simulink model "sh_water_supply_system"  (R2019a)
settings: Solver=VariableStepAuto  StartTime=0.0  StopTime=200  MaxStep=0.1  RelTol=1e-3  EnableMultiTasking=on
PreLoadFcn:
  | sh_water_supply_system_init
libraries: sh_lib x35, fl_lib x12, nesl_utility x11
CloseFcn:
  | try,close(h1_sh_water_supply_system),end
  | clear h1_sh_water_supply_system
  | 
  | 
  | clear simlog_sh_water_supply_system
Description:
  | Water Supply System
  | 
  | Copyright 2008-2019 The MathWorks, Inc.
settings Model: Creator=MathWorks  LastModifiedBy=jaych
settings DataIOCC: LimitDataPoints=on  MaxDataPoints=10000  SaveFormat=Array  SignalLoggingSaveFormat=ModelDataLogs  ReturnWorkspaceOutputs=off  SignalLoggingName=logsout_sh_water_supply_system
settings OptimizationCC: ExpressionDepthLimit=2147483647  LifeSpan=inf
settings DebuggingCC: UnderspecifiedInitializationDetection=Classic  MergeDetectMultiDrivingBlocksExec=none  SolverPrmCheckMsg=warning  FcnCallInpInsideContextMsg=warning  AllowSymbolicDim=off  StateNameClashWarn=warning  PregeneratedLibrarySubsystemCodeDiagnostic=none  SFUnexpectedBacktrackingDiag=warning  SFNoUnconditionalDefaultTransitionDiag=warning  SFExecutionAtInitializationDiag=none  ArithmeticOperatorsInVariantConditions=warning
settings HardwareCC: ProdBitPerPointer=32  ProdBitPerSizeT=32  ProdBitPerPtrDiffT=32  ProdLargestAtomicFloat=None  ProdIntDivRoundTo=Undefined  ProdEndianess=Unspecified  ProdWordSize=32  ProdHWDeviceType=32-bit Generic
settings ModelReferenceCC: PropagateSignalLabelsOutOfModel=off
settings SFSimCC: SimUseLocalCustomCode=off
settings RTWCC: RTWUseLocalCustomCode=off
settings CodeAppCC: StateflowObjectComments=on
settings GRTTargetCC: TargetLangStandard=C89/C90 (ANSI)  GeneratePreprocessorConditionals=Disable all  CombineOutputUpdateFcns=off  GRTInterface=on
settings ConfigComp: CovMetricSettings=dw  CovHtmlReporting=on  CovSaveCumulativeToWorkspaceVar=on  CovSaveSingleToWorkspaceVar=on  CovExternalEMLEnable=off  CovSFcnEnable=off
settings SimscapeCC: SimscapeLogType=all  SimscapeLogSimulationStatistics=on  SimscapeLogName=simlog_sh_water_supply_system  SimscapeLogDataHistory=10000

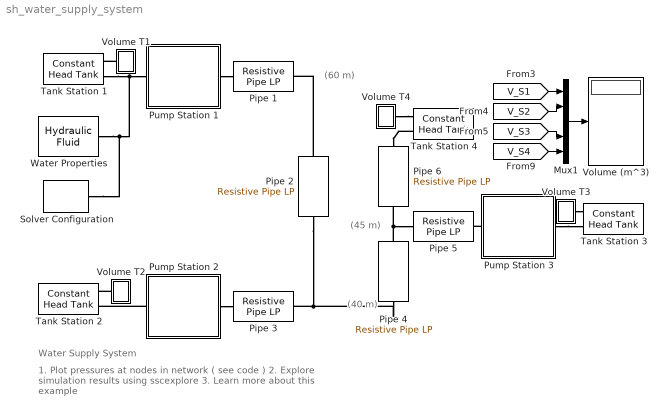
== system sh_water_supply_system ==
  note: (60 m)
  note: (40 m)
  note: (45 m)
  note: Water Supply System
  note: 1. Plot pressures at nodes in network ( see code )
      | 2. Explore simulation results using sscexplore
      | 3. Learn more about this example
  Mux1 : Mux  Inputs=5
  Pipe 1 : sh_lib/Low-Pressure Blocks/Resistive Pipe LP  cs_type=1  d_in=LP_1.diameter mm  area=1e-04 m^2  D_h=0.0112 m  s_factor=64  length=LP_1.length m  length_ad=1 m  roughness=0.005 mm  Re_lam=2e+03  Re_turb=4e+03  elevation_A=LP_1.elevation_A m  elevation_B=LP_1.elevation_B m  g=9.80665 m/s^2  pressure_drop_specify=off  pressure_drop_priority=None  pressure_drop=0 Pa  pressure_drop_nominal_specify=off  pressure_drop_nominal_unit=Pa  pressure_drop_nominal_value=1  flow_rate_specify=off  flow_rate_priority=None  flow_rate=0 m^3/s  flow_rate_nominal_specify=off  flow_rate_nominal_unit=m^3/s  flow_rate_nominal_value=1
      settings: SourceProductName=Simscape Fluids  SourceProductBaseCode=SH
  Pipe 2 : sh_lib/Low-Pressure Blocks/Resistive Pipe LP  cs_type=1  d_in=LP_2.diameter mm  area=1e-04 m^2  D_h=0.0112 m  s_factor=64  length=LP_2.length m  length_ad=1 m  roughness=0.005 mm  Re_lam=2e+03  Re_turb=4e+03  elevation_A=LP_2.elevation_A m  elevation_B=LP_2.elevation_B m  g=9.80665 m/s^2  pressure_drop_specify=off  pressure_drop_priority=None  pressure_drop=0 Pa  pressure_drop_nominal_specify=off  pressure_drop_nominal_unit=Pa  pressure_drop_nominal_value=1  flow_rate_specify=off  flow_rate_priority=None  flow_rate=0 m^3/s  flow_rate_nominal_specify=off  flow_rate_nominal_unit=m^3/s  flow_rate_nominal_value=1
      settings: SourceProductName=Simscape Fluids  SourceProductBaseCode=SH
  Pipe 3 : sh_lib/Low-Pressure Blocks/Resistive Pipe LP  cs_type=1  d_in=LP_3.diameter mm  area=1e-04 m^2  D_h=0.0112 m  s_factor=64  length=LP_3.length m  length_ad=1 m  roughness=0.005 mm  Re_lam=2e+03  Re_turb=4e+03  elevation_A=LP_3.elevation_A m  elevation_B=LP_3.elevation_B m  g=9.80665 m/s^2  pressure_drop_specify=off  pressure_drop_priority=None  pressure_drop=0 Pa  pressure_drop_nominal_specify=off  pressure_drop_nominal_unit=Pa  pressure_drop_nominal_value=1  flow_rate_specify=off  flow_rate_priority=None  flow_rate=0 m^3/s  flow_rate_nominal_specify=off  flow_rate_nominal_unit=m^3/s  flow_rate_nominal_value=1
      settings: SourceProductName=Simscape Fluids  SourceProductBaseCode=SH
  Pipe 4 : sh_lib/Low-Pressure Blocks/Resistive Pipe LP  cs_type=1  d_in=LP_4.diameter mm  area=1e-04 m^2  D_h=0.0112 m  s_factor=64  length=LP_4.length m  length_ad=1 m  roughness=0.005 mm  Re_lam=2e+03  Re_turb=4e+03  elevation_A=LP_4.elevation_A m  elevation_B=LP_4.elevation_B m  g=9.80665 m/s^2  pressure_drop_specify=off  pressure_drop_priority=None  pressure_drop=0 Pa  pressure_drop_nominal_specify=off  pressure_drop_nominal_unit=Pa  pressure_drop_nominal_value=1  flow_rate_specify=off  flow_rate_priority=None  flow_rate=0 m^3/s  flow_rate_nominal_specify=off  flow_rate_nominal_unit=m^3/s  flow_rate_nominal_value=1
      settings: SourceProductName=Simscape Fluids  SourceProductBaseCode=SH
  Pipe 5 : sh_lib/Low-Pressure Blocks/Resistive Pipe LP  cs_type=1  d_in=LP_5.diameter mm  area=1e-04 m^2  D_h=0.0112 m  s_factor=64  length=LP_5.length m  length_ad=1 m  roughness=0.005 mm  Re_lam=2e+03  Re_turb=4e+03  elevation_A=LP_5.elevation_A m  elevation_B=LP_5.elevation_B m  g=9.80665 m/s^2  pressure_drop_specify=off  pressure_drop_priority=None  pressure_drop=0 Pa  pressure_drop_nominal_specify=off  pressure_drop_nominal_unit=Pa  pressure_drop_nominal_value=1  flow_rate_specify=off  flow_rate_priority=None  flow_rate=0 m^3/s  flow_rate_nominal_specify=off  flow_rate_nominal_unit=m^3/s  flow_rate_nominal_value=1
      settings: SourceProductName=Simscape Fluids  SourceProductBaseCode=SH
  Pipe 6 : sh_lib/Low-Pressure Blocks/Resistive Pipe LP  cs_type=1  d_in=LP_6.diameter mm  area=1e-04 m^2  D_h=0.0112 m  s_factor=64  length=LP_6.length m  length_ad=1 m  roughness=0.005 mm  Re_lam=2e+03  Re_turb=4e+03  elevation_A=LP_6.elevation_A m  elevation_B=LP_6.elevation_B m  g=9.80665 m/s^2  pressure_drop_specify=off  pressure_drop_priority=None  pressure_drop=0 Pa  pressure_drop_nominal_specify=off  pressure_drop_nominal_unit=Pa  pressure_drop_nominal_value=1  flow_rate_specify=off  flow_rate_priority=None  flow_rate=0 m^3/s  flow_rate_nominal_specify=off  flow_rate_nominal_unit=m^3/s  flow_rate_nominal_value=1
      settings: SourceProductName=Simscape Fluids  SourceProductBaseCode=SH
  Pump Station 1 : Subsystem  Tag=PublishSubsystem
      mask Display:
      | plot(sin(0:0.5:4.5*pi)*0.9, cos(0:0.5:4.5*pi)*0.9+1.5)
      | plot(sin(0:0.5:4.5*pi)*0.5, cos(0:0.5:4.5*pi)*0.5+1.5)
      | plot(sin(0:0.5:4.5*pi)*0.9, cos(0:0.5:4.5*pi)*0.9-1.5)
      | plot(sin(0:0.5:4.5*pi)*0.5, cos(0:0.5:4.5*pi)*0.5-1.5)
      | 
      | plot([0 -0.9],[1.5 1.5-0.9])
      | plot([0 -0.9],[1.5 1.5-0.9]*-1)
      | 
      | plot([0.45 0.45 0.325 0.325]*2,[1.5 1.5-1.0 1.5-1.0 1.5-0.55])
      | plot([0.45 0.45 0.325 0.325]*2,[1.5 1.5-0.9 1.5-0.9 1.5-0.55]*-1)
      | 
      | plot([2.2 0.95]*-1,[0 0])
      | plot([2.2 0.95],[0 0])
      | 
      | plot([0.95 0.95]*-1,[-0.6 0.6])
      | plot([0.8 0.8],[-0.55 0.55])
      | 
      | 
      | color('white');plot(-3,-2.5);plot(3,2.5);
      | color('red');
      | port_label('LConn',1,'T');
      | port_label('RConn',1,'P');
  Pump Station 2 : Subsystem
      mask Display:
      | %text(0.1,0.7,'Pump Station 1');
      | %text(0.1,0.3,'Elevation 45 m');
      | plot(sin(0:0.5:4.5*pi)*0.9, cos(0:0.5:4.5*pi)*0.9+1.5)
      | plot(sin(0:0.5:4.5*pi)*0.5, cos(0:0.5:4.5*pi)*0.5+1.5)
      | plot(sin(0:0.5:4.5*pi)*0.9, cos(0:0.5:4.5*pi)*0.9-1.5)
      | plot(sin(0:0.5:4.5*pi)*0.5, cos(0:0.5:4.5*pi)*0.5-1.5)
      | 
      | plot([0 -0.9],[1.5 1.5-0.9])
      | plot([0 -0.9],[1.5 1.5-0.9]*-1)
      | 
      | plot([0.45 0.45 0.325 0.325]*2,[1.5 1.5-1.0 1.5-1.0 1.5-0.55])
      | plot([0.45 0.45 0.325 0.325]*2,[1.5 1.5-0.9 1.5-0.9 1.5-0.55]*-1)
      | 
      | plot([2.2 0.95]*-1,[0 0])
      | plot([2.2 0.95],[0 0])
      | 
      | plot([0.95 0.95]*-1,[-0.6 0.6])
      | plot([0.8 0.8],[-0.55 0.55])
      | 
      | 
      | color('white');plot(-3,-2.5);plot(3,2.5);
      | color('red');
      | port_label('LConn',1,'T');
      | port_label('RConn',1,'P');
  Pump Station 3 : Subsystem
      mask Display:
      | %text(0.1,0.7,'Pump Station 1');
      | %text(0.1,0.3,'Elevation 45 m');
      | plot(sin(0:0.5:4.5*pi)*0.9, cos(0:0.5:4.5*pi)*0.9+1.5)
      | plot(sin(0:0.5:4.5*pi)*0.5, cos(0:0.5:4.5*pi)*0.5+1.5)
      | plot(sin(0:0.5:4.5*pi)*0.9, cos(0:0.5:4.5*pi)*0.9-1.5)
      | plot(sin(0:0.5:4.5*pi)*0.5, cos(0:0.5:4.5*pi)*0.5-1.5)
      | 
      | plot([0 -0.9],[1.5 1.5-0.9])
      | plot([0 -0.9],[1.5 1.5-0.9]*-1)
      | 
      | plot([0.45 0.45 0.325 0.325]*2,[1.5 1.5-1.0 1.5-1.0 1.5-0.55])
      | plot([0.45 0.45 0.325 0.325]*2,[1.5 1.5-0.9 1.5-0.9 1.5-0.55]*-1)
      | 
      | plot([2.2 0.95]*-1,[0 0])
      | plot([2.2 0.95],[0 0])
      | 
      | plot([0.95 0.95]*-1,[-0.6 0.6])
      | plot([0.8 0.8],[-0.55 0.55])
      | 
      | 
      | color('white');plot(-3,-2.5);plot(3,2.5);
      | color('red');
      | port_label('LConn',1,'T');
      | port_label('RConn',1,'P');
  Solver Configuration : nesl_utility/Solver Configuration  PhysicalDomain=network_engine_domain  SubClassName=solver  LeftPortType=input  RightPortType=generic  Tones=[]  Harmonics=[]  SimulateNoise=off  Profile=off  UseLocalSampling=off  EnableSwitchedLinearOptims=on  FrequencyDomain=off  UseCCode=off  RelTol=0.001  AbsTol=1e-06  MinStep=1e-09  ToWorkspace=off  RevertToSquareIcSolve=off  NumHomotopyIterations=100  PhasorMode=off  PhasorModeNumHarmonics=1  DoDC=off  ResidualTolerance=1e-9  UseLocalSolver=off  LocalSolverChoice=NE_BACKWARD_EULER_ADVANCER  LocalSolverSampleTime=.001  DoFixedCost=off  MaxNonlinIter=3  MaxModeIter=2  LinearAlgebra=auto  EquationFormulation=NE_TIME_EF  DelaysMemoryBudget=1024  AutomaticFiltering=on  FilteringTimeConstant=0.001  PartitionStorageMethod=AS_NEEDED  PartitionMemoryBudget=1024  PartitionMethod=FAST
  Tank Station 1 : sh_lib/Low-Pressure Blocks/Constant Head Tank  press=0 Pa  fluid_level=station_1.fluid_level m  pipe_diam=0.02 m  loss_coeff=1.2  g=9.80665 m/s^2  volume_specify=on  volume_priority=High  volume=100 m^3  volume_nominal_specify=off  volume_nominal_unit=m^3  volume_nominal_value=1
      settings: SourceProductName=Simscape Fluids  SourceProductBaseCode=SH
  Tank Station 2 : sh_lib/Low-Pressure Blocks/Constant Head Tank  press=0 Pa  fluid_level=station_2.fluid_level m  pipe_diam=0.02 m  loss_coeff=1.2  g=9.80665 m/s^2  volume_specify=on  volume_priority=High  volume=100 m^3  volume_nominal_specify=off  volume_nominal_unit=m^3  volume_nominal_value=1
      settings: SourceProductName=Simscape Fluids  SourceProductBaseCode=SH
  Tank Station 3 : sh_lib/Low-Pressure Blocks/Constant Head Tank  press=0 Pa  fluid_level=station_3.fluid_level m  pipe_diam=0.02 m  loss_coeff=1.2  g=9.80665 m/s^2  volume_specify=on  volume_priority=High  volume=100 m^3  volume_nominal_specify=off  volume_nominal_unit=m^3  volume_nominal_value=1
      settings: SourceProductName=Simscape Fluids  SourceProductBaseCode=SH
  Tank Station 4 : sh_lib/Low-Pressure Blocks/Constant Head Tank  press=0 Pa  fluid_level=0 m  pipe_diam=0.02 m  loss_coeff=1.2  g=9.80665 m/s^2  volume_specify=on  volume_priority=High  volume=0 m^3  volume_nominal_specify=off  volume_nominal_unit=m^3  volume_nominal_value=1
      settings: SourceProductName=Simscape Fluids  SourceProductBaseCode=SH
  Volume (m^3) : Display
  Volume T1 : Subsystem
  Volume T2 : Subsystem
  Volume T3 : Subsystem
  Volume T4 : Subsystem
  Water Properties : sh_lib/Hydraulic Utilities/Hydraulic Fluid  DataSource=1  SelFluid=24  SysTemp=1  TrapAir=0.001  ViscDerFactor=1  range_error=2
      settings: SourceProductName=Simscape Fluids
  wires:
  [V_S1] -> Mux1/1
  [V_S2] -> Mux1/2
  [V_S3] -> Mux1/4
  Mux1/1 -> Volume (m^3)/1
  [V_S4] -> Mux1/5
  connections:
  Pump Station 1/RConn1 -- Pipe 1/LConn1
  Pipe 2/LConn1 -- Pipe 1/RConn1
  Pump Station 2/RConn1 -- Pipe 3/LConn1
  Pipe 4/LConn1 -- Pipe 2/RConn1 -- Pipe 3/RConn1
  Tank Station 4/RConn2 -- Pipe 6/RConn1
  Pipe 4/RConn1 -- Pipe 5/RConn1 -- Pipe 6/LConn1
  Tank Station 1/RConn2 -- Solver Configuration/RConn1 -- Water Properties/RConn1 -- Pump Station 1/LConn1
  Volume T1/LConn1 -- Tank Station 1/RConn1
  Pump Station 2/LConn1 -- Tank Station 2/RConn2
  Volume T2/LConn1 -- Tank Station 2/RConn1
  Pump Station 3/RConn1 -- Pipe 5/LConn1
  Pump Station 3/LConn1 -- Tank Station 3/RConn2
  Volume T3/LConn1 -- Tank Station 3/RConn1
  Volume T4/LConn1 -- Tank Station 4/RConn1

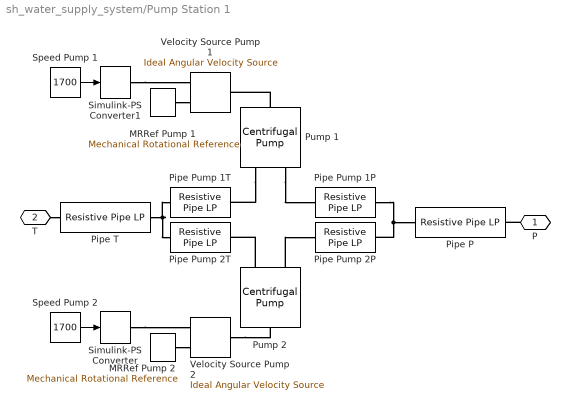
== system sh_water_supply_system/Pump Station 1 ==
  MRRef Pump 1 : fl_lib/Mechanical/Rotational Elements/Mechanical Rotational Reference
  MRRef Pump 2 : fl_lib/Mechanical/Rotational Elements/Mechanical Rotational Reference
  Pipe P : sh_lib/Low-Pressure Blocks/Resistive Pipe LP  cs_type=1  d_in=station_1.pipe_diameter mm  area=1e-04 m^2  D_h=0.0112 m  s_factor=64  length=station_1.pipe_length_3 m  length_ad=1 m  roughness=0.005 mm  Re_lam=2e+03  Re_turb=4e+03  elevation_A=station_1.elevation m  elevation_B=station_1.elevation m  g=9.80665 m/s^2  pressure_drop_specify=off  pressure_drop_priority=None  pressure_drop=0 Pa  pressure_drop_nominal_specify=off  pressure_drop_nominal_unit=Pa  pressure_drop_nominal_value=1  flow_rate_specify=off  flow_rate_priority=None  flow_rate=0 m^3/s  flow_rate_nominal_specify=off  flow_rate_nominal_unit=m^3/s  flow_rate_nominal_value=1
      settings: SourceProductName=Simscape Fluids  SourceProductBaseCode=SH
  Pipe Pump 1P : sh_lib/Low-Pressure Blocks/Resistive Pipe LP  cs_type=1  d_in=station_1.pipe_diameter mm  area=1e-04 m^2  D_h=0.0112 m  s_factor=64  length=station_1.pipe_length_2 m  length_ad=1 m  roughness=0.005 mm  Re_lam=2e+03  Re_turb=4e+03  elevation_A=station_1.elevation m  elevation_B=station_1.elevation m  g=9.80665 m/s^2  pressure_drop_specify=off  pressure_drop_priority=None  pressure_drop=0 Pa  pressure_drop_nominal_specify=off  pressure_drop_nominal_unit=Pa  pressure_drop_nominal_value=1  flow_rate_specify=off  flow_rate_priority=None  flow_rate=0 m^3/s  flow_rate_nominal_specify=off  flow_rate_nominal_unit=m^3/s  flow_rate_nominal_value=1
      settings: SourceProductName=Simscape Fluids  SourceProductBaseCode=SH
  Pipe Pump 1T : sh_lib/Low-Pressure Blocks/Resistive Pipe LP  cs_type=1  d_in=station_1.pipe_diameter mm  area=1e-04 m^2  D_h=0.0112 m  s_factor=64  length=station_1.pipe_length_2 m  length_ad=1 m  roughness=0.005 mm  Re_lam=2e+03  Re_turb=4e+03  elevation_A=station_1.elevation m  elevation_B=station_1.elevation m  g=9.80665 m/s^2  pressure_drop_specify=off  pressure_drop_priority=None  pressure_drop=0 Pa  pressure_drop_nominal_specify=off  pressure_drop_nominal_unit=Pa  pressure_drop_nominal_value=1  flow_rate_specify=off  flow_rate_priority=None  flow_rate=0 m^3/s  flow_rate_nominal_specify=off  flow_rate_nominal_unit=m^3/s  flow_rate_nominal_value=1
      settings: SourceProductName=Simscape Fluids  SourceProductBaseCode=SH
  Pipe Pump 2P : sh_lib/Low-Pressure Blocks/Resistive Pipe LP  cs_type=1  d_in=station_1.pipe_diameter mm  area=1e-04 m^2  D_h=0.0112 m  s_factor=64  length=station_1.pipe_length_2 m  length_ad=1 m  roughness=0.005 mm  Re_lam=2e+03  Re_turb=4e+03  elevation_A=station_1.elevation m  elevation_B=station_1.elevation m  g=9.80665 m/s^2  pressure_drop_specify=off  pressure_drop_priority=None  pressure_drop=0 Pa  pressure_drop_nominal_specify=off  pressure_drop_nominal_unit=Pa  pressure_drop_nominal_value=1  flow_rate_specify=off  flow_rate_priority=None  flow_rate=0 m^3/s  flow_rate_nominal_specify=off  flow_rate_nominal_unit=m^3/s  flow_rate_nominal_value=1
      settings: SourceProductName=Simscape Fluids  SourceProductBaseCode=SH
  Pipe Pump 2T : sh_lib/Low-Pressure Blocks/Resistive Pipe LP  cs_type=1  d_in=station_1.pipe_diameter mm  area=1e-04 m^2  D_h=0.0112 m  s_factor=64  length=station_1.pipe_length_2 m  length_ad=1 m  roughness=0.005 mm  Re_lam=2e+03  Re_turb=4e+03  elevation_A=station_1.elevation m  elevation_B=station_1.elevation m  g=9.80665 m/s^2  pressure_drop_specify=off  pressure_drop_priority=None  pressure_drop=0 Pa  pressure_drop_nominal_specify=off  pressure_drop_nominal_unit=Pa  pressure_drop_nominal_value=1  flow_rate_specify=off  flow_rate_priority=None  flow_rate=0 m^3/s  flow_rate_nominal_specify=off  flow_rate_nominal_unit=m^3/s  flow_rate_nominal_value=1
      settings: SourceProductName=Simscape Fluids  SourceProductBaseCode=SH
  Pipe T : sh_lib/Low-Pressure Blocks/Resistive Pipe LP  cs_type=1  d_in=station_1.pipe_diameter mm  area=1e-04 m^2  D_h=0.0112 m  s_factor=64  length=station_1.pipe_length_1 m  length_ad=1 m  roughness=0.005 mm  Re_lam=2e+03  Re_turb=4e+03  elevation_A=station_1.elevation m  elevation_B=station_1.elevation m  g=9.80665 m/s^2  pressure_drop_specify=off  pressure_drop_priority=None  pressure_drop=0 Pa  pressure_drop_nominal_specify=off  pressure_drop_nominal_unit=Pa  pressure_drop_nominal_value=1  flow_rate_specify=off  flow_rate_priority=None  flow_rate=0 m^3/s  flow_rate_nominal_specify=off  flow_rate_nominal_unit=m^3/s  flow_rate_nominal_value=1
      settings: SourceProductName=Simscape Fluids  SourceProductBaseCode=SH
  Pump 1 : sh_lib/Pumps and Motors/Centrifugal Pump  mdl_type=2  c_1=326.8 Pa/(kg/m^3)  c_2=3.104e+04 Pa*s/kg  c_3=1.097e+07 Pa*s^2/(kg*m^3)  c_4=2.136e+05 Pa*s^2/(kg*m^3)  c_f=0.8  design_del=130 lpm  ref_velocity=1.77e+03 rpm  ref_density=1000 kg/m^3  leak_resistance=1e+8 Pa/(m^3/s)  T_const=0.1 N*m  trq_press_coeff=1e-6 N*m/Pa  pump_del_1D=pump_1.Q m^3/s  press_diff_1D=pump_1.P bar  pump_del_power_1D=pump_1.Q m^3/s  power_1D=pump_1.N W  pump_vel_2D="[  3.2e+03 3.3e+03 3.4e+03 3.5e+03 ] rpm"  pump_del_2D="[  0 50 100 150 200 250 300 350 ] lpm"  press_diff_2D="[  8.3 8.8 9.3 9.9 ; 7.8 8.3 8.8 9.4 ; 7.2 7.6 8.2 8.7 ; 6.5 7 7.5 8 ; 5.6 6.1 6.6 7.1 ; 4.7 5.2 5.7 6.2 ; 3.4 4 4.4 4.9 ; 2.3 2.7 3.4 3.6 ; ] bar"  pump_del_power_2D="[  0 50 100 150 200 250 300 350 ] lpm"  power_2D="[  1.223e+03 1.341e+03 1.467e+03 1.6e+03 ; 1.414e+03 1.551e+03 1.696e+03 1.85e+03 ; 1.636e+03 1.794e+03 1.962e+03 2.14e+03 ; 1.941e+03 2.129e+03 2.326e+03 2.54e+03 ; 2.224e+03 2.439e+03 2.66e+03 2.91e+03 ; 2.453e+03 2.691e+03 2.947e+03 3.21e+03 ; 2.757e+03 3.024e+03 3.307e+03 3.608e+03 ; 2.945e+03 3.23e+03 3.533e+03 3.854e+03 ; ] W"  omega_threshold=1e-9 rad/s  interp_method=2  extrap_method=1
      settings: SourceProductName=Simscape Fluids  SourceProductBaseCode=SH
  Pump 2 : sh_lib/Pumps and Motors/Centrifugal Pump  mdl_type=2  c_1=326.8 Pa/(kg/m^3)  c_2=3.104e+04 Pa*s/kg  c_3=1.097e+07 Pa*s^2/(kg*m^3)  c_4=2.136e+05 Pa*s^2/(kg*m^3)  c_f=0.8  design_del=130 lpm  ref_velocity=1.77e+03 rpm  ref_density=1000 kg/m^3  leak_resistance=1e+8 Pa/(m^3/s)  T_const=0.1 N*m  trq_press_coeff=1e-6 N*m/Pa  pump_del_1D=pump_1.Q m^3/s  press_diff_1D=pump_1.P bar  pump_del_power_1D=pump_1.Q m^3/s  power_1D=pump_1.N W  pump_vel_2D="[  3.2e+03 3.3e+03 3.4e+03 3.5e+03 ] rpm"  pump_del_2D="[  0 50 100 150 200 250 300 350 ] lpm"  press_diff_2D="[  8.3 8.8 9.3 9.9 ; 7.8 8.3 8.8 9.4 ; 7.2 7.6 8.2 8.7 ; 6.5 7 7.5 8 ; 5.6 6.1 6.6 7.1 ; 4.7 5.2 5.7 6.2 ; 3.4 4 4.4 4.9 ; 2.3 2.7 3.4 3.6 ; ] bar"  pump_del_power_2D="[  0 50 100 150 200 250 300 350 ] lpm"  power_2D="[  1.223e+03 1.341e+03 1.467e+03 1.6e+03 ; 1.414e+03 1.551e+03 1.696e+03 1.85e+03 ; 1.636e+03 1.794e+03 1.962e+03 2.14e+03 ; 1.941e+03 2.129e+03 2.326e+03 2.54e+03 ; 2.224e+03 2.439e+03 2.66e+03 2.91e+03 ; 2.453e+03 2.691e+03 2.947e+03 3.21e+03 ; 2.757e+03 3.024e+03 3.307e+03 3.608e+03 ; 2.945e+03 3.23e+03 3.533e+03 3.854e+03 ; ] W"  omega_threshold=1e-9 rad/s  interp_method=2  extrap_method=1
      settings: SourceProductName=Simscape Fluids  SourceProductBaseCode=SH
  Simulink-PS Converter : nesl_utility/Simulink-PS Converter  PhysicalDomain=network_engine_domain  SubClassName=ps_input  LeftPortType=input  RightPortType=output  PseudoPeriodic=off  Frequencies=[]  NoiseDistribution=none  NoiseParameters=[]  Unit=rpm  AffineConversion=off  FilteringAndDerivatives=zero  SimscapeFilterOrder=1  InputFilterTimeConstant=.001  UdotUserProvided=0
  Simulink-PS Converter1 : nesl_utility/Simulink-PS Converter  PhysicalDomain=network_engine_domain  SubClassName=ps_input  LeftPortType=input  RightPortType=output  PseudoPeriodic=off  Frequencies=[]  NoiseDistribution=none  NoiseParameters=[]  Unit=rpm  AffineConversion=off  FilteringAndDerivatives=zero  SimscapeFilterOrder=1  InputFilterTimeConstant=.001  UdotUserProvided=0
  Speed Pump 1 : Constant  Value=1700
  Speed Pump 2 : Constant  Value=1700
  Velocity Source Pump 1 : fl_lib/Mechanical/Mechanical Sources/Ideal Angular Velocity Source
  Velocity Source Pump 2 : fl_lib/Mechanical/Mechanical Sources/Ideal Angular Velocity Source
  P : PMIOPort  Side=Right
  T : PMIOPort  Port=2  Side=Left
  wires:
  Speed Pump 2/1 -> Simulink-PS Converter/1
  Speed Pump 1/1 -> Simulink-PS Converter1/1
  connections:
  Velocity Source Pump 2/LConn1 -- Pump 2/LConn1
  Pump 1/RConn1 -- Pipe Pump 1P/LConn1
  Pump 1/RConn2 -- Pipe Pump 1T/RConn1
  Pump 2/RConn2 -- Pipe Pump 2T/RConn1
  T/RConn1 -- Pipe T/LConn1
  Pump 2/RConn1 -- Pipe Pump 2P/LConn1
  Pipe T/RConn1 -- Pipe Pump 2T/LConn1 -- Pipe Pump 1T/LConn1
  Simulink-PS Converter/RConn1 -- Velocity Source Pump 2/RConn1
  MRRef Pump 2/LConn1 -- Velocity Source Pump 2/RConn2
  Pipe Pump 1P/RConn1 -- Pipe Pump 2P/RConn1 -- Pipe P/LConn1
  P/RConn1 -- Pipe P/RConn1
  MRRef Pump 1/LConn1 -- Velocity Source Pump 1/RConn2
  Pump 1/LConn1 -- Velocity Source Pump 1/LConn1
  Simulink-PS Converter1/RConn1 -- Velocity Source Pump 1/RConn1

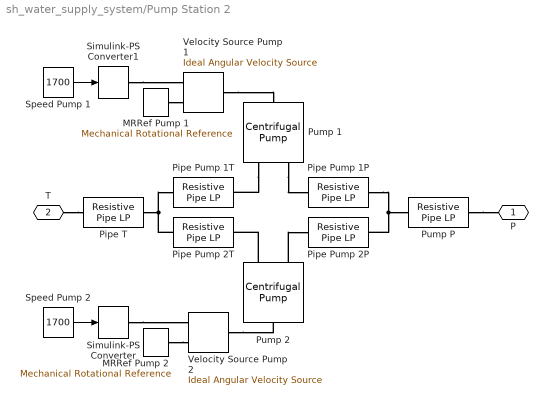
== system sh_water_supply_system/Pump Station 2 ==
  MRRef Pump 1 : fl_lib/Mechanical/Rotational Elements/Mechanical Rotational Reference
  MRRef Pump 2 : fl_lib/Mechanical/Rotational Elements/Mechanical Rotational Reference
  Pipe Pump 1P : sh_lib/Low-Pressure Blocks/Resistive Pipe LP  cs_type=1  d_in=station_2.pipe_diameter mm  area=1e-04 m^2  D_h=0.0112 m  s_factor=64  length=station_2.pipe_length_2 m  length_ad=1 m  roughness=0.005 mm  Re_lam=2e+03  Re_turb=4e+03  elevation_A=station_2.elevation m  elevation_B=station_2.elevation m  g=9.80665 m/s^2  pressure_drop_specify=off  pressure_drop_priority=None  pressure_drop=0 Pa  pressure_drop_nominal_specify=off  pressure_drop_nominal_unit=Pa  pressure_drop_nominal_value=1  flow_rate_specify=off  flow_rate_priority=None  flow_rate=0 m^3/s  flow_rate_nominal_specify=off  flow_rate_nominal_unit=m^3/s  flow_rate_nominal_value=1
      settings: SourceProductName=Simscape Fluids  SourceProductBaseCode=SH
  Pipe Pump 1T : sh_lib/Low-Pressure Blocks/Resistive Pipe LP  cs_type=1  d_in=station_2.pipe_diameter mm  area=1e-04 m^2  D_h=0.0112 m  s_factor=64  length=station_2.pipe_length_2 m  length_ad=1 m  roughness=0.005 mm  Re_lam=2e+03  Re_turb=4e+03  elevation_A=station_2.elevation m  elevation_B=station_2.elevation m  g=9.80665 m/s^2  pressure_drop_specify=off  pressure_drop_priority=None  pressure_drop=0 Pa  pressure_drop_nominal_specify=off  pressure_drop_nominal_unit=Pa  pressure_drop_nominal_value=1  flow_rate_specify=off  flow_rate_priority=None  flow_rate=0 m^3/s  flow_rate_nominal_specify=off  flow_rate_nominal_unit=m^3/s  flow_rate_nominal_value=1
      settings: SourceProductName=Simscape Fluids  SourceProductBaseCode=SH
  Pipe Pump 2P : sh_lib/Low-Pressure Blocks/Resistive Pipe LP  cs_type=1  d_in=station_2.pipe_diameter mm  area=1e-04 m^2  D_h=0.0112 m  s_factor=64  length=station_2.pipe_length_2 m  length_ad=1 m  roughness=0.005 mm  Re_lam=2e+03  Re_turb=4e+03  elevation_A=station_2.elevation m  elevation_B=station_2.elevation m  g=9.80665 m/s^2  pressure_drop_specify=off  pressure_drop_priority=None  pressure_drop=0 Pa  pressure_drop_nominal_specify=off  pressure_drop_nominal_unit=Pa  pressure_drop_nominal_value=1  flow_rate_specify=off  flow_rate_priority=None  flow_rate=0 m^3/s  flow_rate_nominal_specify=off  flow_rate_nominal_unit=m^3/s  flow_rate_nominal_value=1
      settings: SourceProductName=Simscape Fluids  SourceProductBaseCode=SH
  Pipe Pump 2T : sh_lib/Low-Pressure Blocks/Resistive Pipe LP  cs_type=1  d_in=station_2.pipe_diameter mm  area=1e-04 m^2  D_h=0.0112 m  s_factor=64  length=station_2.pipe_length_2 m  length_ad=1 m  roughness=0.005 mm  Re_lam=2e+03  Re_turb=4e+03  elevation_A=station_2.elevation m  elevation_B=station_2.elevation m  g=9.80665 m/s^2  pressure_drop_specify=off  pressure_drop_priority=None  pressure_drop=0 Pa  pressure_drop_nominal_specify=off  pressure_drop_nominal_unit=Pa  pressure_drop_nominal_value=1  flow_rate_specify=off  flow_rate_priority=None  flow_rate=0 m^3/s  flow_rate_nominal_specify=off  flow_rate_nominal_unit=m^3/s  flow_rate_nominal_value=1
      settings: SourceProductName=Simscape Fluids  SourceProductBaseCode=SH
  Pipe T : sh_lib/Low-Pressure Blocks/Resistive Pipe LP  cs_type=1  d_in=station_2.pipe_diameter mm  area=1e-04 m^2  D_h=0.0112 m  s_factor=64  length=station_2.pipe_length_1 m  length_ad=1 m  roughness=0.005 mm  Re_lam=2e+03  Re_turb=4e+03  elevation_A=station_2.elevation m  elevation_B=station_2.elevation m  g=9.80665 m/s^2  pressure_drop_specify=off  pressure_drop_priority=None  pressure_drop=0 Pa  pressure_drop_nominal_specify=off  pressure_drop_nominal_unit=Pa  pressure_drop_nominal_value=1  flow_rate_specify=off  flow_rate_priority=None  flow_rate=0 m^3/s  flow_rate_nominal_specify=off  flow_rate_nominal_unit=m^3/s  flow_rate_nominal_value=1
      settings: SourceProductName=Simscape Fluids  SourceProductBaseCode=SH
  Pump 1 : sh_lib/Pumps and Motors/Centrifugal Pump  mdl_type=2  c_1=326.8 Pa/(kg/m^3)  c_2=3.104e+04 Pa*s/kg  c_3=1.097e+07 Pa*s^2/(kg*m^3)  c_4=2.136e+05 Pa*s^2/(kg*m^3)  c_f=0.8  design_del=130 lpm  ref_velocity=1.77e+03 rpm  ref_density=1000 kg/m^3  leak_resistance=1e+8 Pa/(m^3/s)  T_const=0.1 N*m  trq_press_coeff=1e-6 N*m/Pa  pump_del_1D=pump_2.Q m^3/s  press_diff_1D=pump_2.P bar  pump_del_power_1D=pump_2.Q m^3/s  power_1D=pump_2.N W  pump_vel_2D="[  3.2e+03 3.3e+03 3.4e+03 3.5e+03 ] rpm"  pump_del_2D="[  0 50 100 150 200 250 300 350 ] lpm"  press_diff_2D="[  8.3 8.8 9.3 9.9 ; 7.8 8.3 8.8 9.4 ; 7.2 7.6 8.2 8.7 ; 6.5 7 7.5 8 ; 5.6 6.1 6.6 7.1 ; 4.7 5.2 5.7 6.2 ; 3.4 4 4.4 4.9 ; 2.3 2.7 3.4 3.6 ; ] bar"  pump_del_power_2D="[  0 50 100 150 200 250 300 350 ] lpm"  power_2D="[  1.223e+03 1.341e+03 1.467e+03 1.6e+03 ; 1.414e+03 1.551e+03 1.696e+03 1.85e+03 ; 1.636e+03 1.794e+03 1.962e+03 2.14e+03 ; 1.941e+03 2.129e+03 2.326e+03 2.54e+03 ; 2.224e+03 2.439e+03 2.66e+03 2.91e+03 ; 2.453e+03 2.691e+03 2.947e+03 3.21e+03 ; 2.757e+03 3.024e+03 3.307e+03 3.608e+03 ; 2.945e+03 3.23e+03 3.533e+03 3.854e+03 ; ] W"  omega_threshold=1e-9 rad/s  interp_method=2  extrap_method=1
      settings: SourceProductName=Simscape Fluids  SourceProductBaseCode=SH
  Pump 2 : sh_lib/Pumps and Motors/Centrifugal Pump  mdl_type=2  c_1=326.8 Pa/(kg/m^3)  c_2=3.104e+04 Pa*s/kg  c_3=1.097e+07 Pa*s^2/(kg*m^3)  c_4=2.136e+05 Pa*s^2/(kg*m^3)  c_f=0.8  design_del=130 lpm  ref_velocity=1.77e+03 rpm  ref_density=1000 kg/m^3  leak_resistance=1e+8 Pa/(m^3/s)  T_const=0.1 N*m  trq_press_coeff=1e-6 N*m/Pa  pump_del_1D=pump_2.Q m^3/s  press_diff_1D=pump_2.P bar  pump_del_power_1D=pump_2.Q m^3/s  power_1D=pump_2.N W  pump_vel_2D="[  3.2e+03 3.3e+03 3.4e+03 3.5e+03 ] rpm"  pump_del_2D="[  0 50 100 150 200 250 300 350 ] lpm"  press_diff_2D="[  8.3 8.8 9.3 9.9 ; 7.8 8.3 8.8 9.4 ; 7.2 7.6 8.2 8.7 ; 6.5 7 7.5 8 ; 5.6 6.1 6.6 7.1 ; 4.7 5.2 5.7 6.2 ; 3.4 4 4.4 4.9 ; 2.3 2.7 3.4 3.6 ; ] bar"  pump_del_power_2D="[  0 50 100 150 200 250 300 350 ] lpm"  power_2D="[  1.223e+03 1.341e+03 1.467e+03 1.6e+03 ; 1.414e+03 1.551e+03 1.696e+03 1.85e+03 ; 1.636e+03 1.794e+03 1.962e+03 2.14e+03 ; 1.941e+03 2.129e+03 2.326e+03 2.54e+03 ; 2.224e+03 2.439e+03 2.66e+03 2.91e+03 ; 2.453e+03 2.691e+03 2.947e+03 3.21e+03 ; 2.757e+03 3.024e+03 3.307e+03 3.608e+03 ; 2.945e+03 3.23e+03 3.533e+03 3.854e+03 ; ] W"  omega_threshold=1e-9 rad/s  interp_method=2  extrap_method=1
      settings: SourceProductName=Simscape Fluids  SourceProductBaseCode=SH
  Pump P : sh_lib/Low-Pressure Blocks/Resistive Pipe LP  cs_type=1  d_in=station_2.pipe_diameter mm  area=1e-04 m^2  D_h=0.0112 m  s_factor=64  length=station_2.pipe_length_3 m  length_ad=1 m  roughness=0.005 mm  Re_lam=2e+03  Re_turb=4e+03  elevation_A=station_2.elevation m  elevation_B=station_2.elevation m  g=9.80665 m/s^2  pressure_drop_specify=off  pressure_drop_priority=None  pressure_drop=0 Pa  pressure_drop_nominal_specify=off  pressure_drop_nominal_unit=Pa  pressure_drop_nominal_value=1  flow_rate_specify=off  flow_rate_priority=None  flow_rate=0 m^3/s  flow_rate_nominal_specify=off  flow_rate_nominal_unit=m^3/s  flow_rate_nominal_value=1
      settings: SourceProductName=Simscape Fluids  SourceProductBaseCode=SH
  Simulink-PS Converter : nesl_utility/Simulink-PS Converter  PhysicalDomain=network_engine_domain  SubClassName=ps_input  LeftPortType=input  RightPortType=output  PseudoPeriodic=off  Frequencies=[]  NoiseDistribution=none  NoiseParameters=[]  Unit=rpm  AffineConversion=off  FilteringAndDerivatives=zero  SimscapeFilterOrder=1  InputFilterTimeConstant=.001  UdotUserProvided=0
  Simulink-PS Converter1 : nesl_utility/Simulink-PS Converter  PhysicalDomain=network_engine_domain  SubClassName=ps_input  LeftPortType=input  RightPortType=output  PseudoPeriodic=off  Frequencies=[]  NoiseDistribution=none  NoiseParameters=[]  Unit=rpm  AffineConversion=off  FilteringAndDerivatives=zero  SimscapeFilterOrder=1  InputFilterTimeConstant=.001  UdotUserProvided=0
  Speed Pump 1 : Constant  Value=1700
  Speed Pump 2 : Constant  Value=1700
  Velocity Source Pump 1 : fl_lib/Mechanical/Mechanical Sources/Ideal Angular Velocity Source
  Velocity Source Pump 2 : fl_lib/Mechanical/Mechanical Sources/Ideal Angular Velocity Source
  P : PMIOPort  Side=Right
  T : PMIOPort  Port=2  Side=Left
  wires:
  Speed Pump 2/1 -> Simulink-PS Converter/1
  Speed Pump 1/1 -> Simulink-PS Converter1/1
  connections:
  Pipe Pump 1P/RConn1 -- Pipe Pump 2P/RConn1 -- Pump P/LConn1
  MRRef Pump 2/LConn1 -- Velocity Source Pump 2/RConn2
  Simulink-PS Converter/RConn1 -- Velocity Source Pump 2/RConn1
  Pipe Pump 2T/LConn1 -- Pipe T/RConn1 -- Pipe Pump 1T/LConn1
  Pump 2/RConn1 -- Pipe Pump 2P/LConn1
  T/RConn1 -- Pipe T/LConn1
  Pump 2/RConn2 -- Pipe Pump 2T/RConn1
  Pump 1/RConn2 -- Pipe Pump 1T/RConn1
  Pump 1/RConn1 -- Pipe Pump 1P/LConn1
  Velocity Source Pump 2/LConn1 -- Pump 2/LConn1
  Pump P/RConn1 -- P/RConn1
  Velocity Source Pump 1/LConn1 -- Pump 1/LConn1
  MRRef Pump 1/LConn1 -- Velocity Source Pump 1/RConn2
  Simulink-PS Converter1/RConn1 -- Velocity Source Pump 1/RConn1

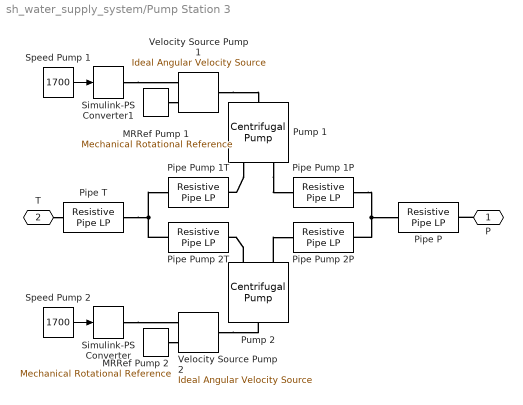
== system sh_water_supply_system/Pump Station 3 ==
  MRRef Pump 1 : fl_lib/Mechanical/Rotational Elements/Mechanical Rotational Reference
  MRRef Pump 2 : fl_lib/Mechanical/Rotational Elements/Mechanical Rotational Reference
  Pipe P : sh_lib/Low-Pressure Blocks/Resistive Pipe LP  cs_type=1  d_in=station_3.pipe_diameter mm  area=1e-04 m^2  D_h=0.0112 m  s_factor=64  length=station_3.pipe_length_3 m  length_ad=1 m  roughness=0.005 mm  Re_lam=2e+03  Re_turb=4e+03  elevation_A=station_3.elevation m  elevation_B=station_3.elevation m  g=9.80665 m/s^2  pressure_drop_specify=off  pressure_drop_priority=None  pressure_drop=0 Pa  pressure_drop_nominal_specify=off  pressure_drop_nominal_unit=Pa  pressure_drop_nominal_value=1  flow_rate_specify=off  flow_rate_priority=None  flow_rate=0 m^3/s  flow_rate_nominal_specify=off  flow_rate_nominal_unit=m^3/s  flow_rate_nominal_value=1
      settings: SourceProductName=Simscape Fluids  SourceProductBaseCode=SH
  Pipe Pump 1P : sh_lib/Low-Pressure Blocks/Resistive Pipe LP  cs_type=1  d_in=station_3.pipe_diameter mm  area=1e-04 m^2  D_h=0.0112 m  s_factor=64  length=station_3.pipe_length_2 m  length_ad=1 m  roughness=0.005 mm  Re_lam=2e+03  Re_turb=4e+03  elevation_A=station_3.elevation m  elevation_B=station_3.elevation m  g=9.80665 m/s^2  pressure_drop_specify=off  pressure_drop_priority=None  pressure_drop=0 Pa  pressure_drop_nominal_specify=off  pressure_drop_nominal_unit=Pa  pressure_drop_nominal_value=1  flow_rate_specify=off  flow_rate_priority=None  flow_rate=0 m^3/s  flow_rate_nominal_specify=off  flow_rate_nominal_unit=m^3/s  flow_rate_nominal_value=1
      settings: SourceProductName=Simscape Fluids  SourceProductBaseCode=SH
  Pipe Pump 1T : sh_lib/Low-Pressure Blocks/Resistive Pipe LP  cs_type=1  d_in=station_3.pipe_diameter mm  area=1e-04 m^2  D_h=0.0112 m  s_factor=64  length=station_3.pipe_length_2 m  length_ad=1 m  roughness=0.005 mm  Re_lam=2e+03  Re_turb=4e+03  elevation_A=station_3.elevation m  elevation_B=station_3.elevation m  g=9.80665 m/s^2  pressure_drop_specify=off  pressure_drop_priority=None  pressure_drop=0 Pa  pressure_drop_nominal_specify=off  pressure_drop_nominal_unit=Pa  pressure_drop_nominal_value=1  flow_rate_specify=off  flow_rate_priority=None  flow_rate=0 m^3/s  flow_rate_nominal_specify=off  flow_rate_nominal_unit=m^3/s  flow_rate_nominal_value=1
      settings: SourceProductName=Simscape Fluids  SourceProductBaseCode=SH
  Pipe Pump 2P : sh_lib/Low-Pressure Blocks/Resistive Pipe LP  cs_type=1  d_in=station_3.pipe_diameter mm  area=1e-04 m^2  D_h=0.0112 m  s_factor=64  length=station_3.pipe_length_2 m  length_ad=1 m  roughness=0.005 mm  Re_lam=2e+03  Re_turb=4e+03  elevation_A=station_3.elevation m  elevation_B=station_3.elevation m  g=9.80665 m/s^2  pressure_drop_specify=off  pressure_drop_priority=None  pressure_drop=0 Pa  pressure_drop_nominal_specify=off  pressure_drop_nominal_unit=Pa  pressure_drop_nominal_value=1  flow_rate_specify=off  flow_rate_priority=None  flow_rate=0 m^3/s  flow_rate_nominal_specify=off  flow_rate_nominal_unit=m^3/s  flow_rate_nominal_value=1
      settings: SourceProductName=Simscape Fluids  SourceProductBaseCode=SH
  Pipe Pump 2T : sh_lib/Low-Pressure Blocks/Resistive Pipe LP  cs_type=1  d_in=station_3.pipe_diameter mm  area=1e-04 m^2  D_h=0.0112 m  s_factor=64  length=station_3.pipe_length_2 m  length_ad=1 m  roughness=0.005 mm  Re_lam=2e+03  Re_turb=4e+03  elevation_A=station_3.elevation m  elevation_B=station_3.elevation m  g=9.80665 m/s^2  pressure_drop_specify=off  pressure_drop_priority=None  pressure_drop=0 Pa  pressure_drop_nominal_specify=off  pressure_drop_nominal_unit=Pa  pressure_drop_nominal_value=1  flow_rate_specify=off  flow_rate_priority=None  flow_rate=0 m^3/s  flow_rate_nominal_specify=off  flow_rate_nominal_unit=m^3/s  flow_rate_nominal_value=1
      settings: SourceProductName=Simscape Fluids  SourceProductBaseCode=SH
  Pipe T : sh_lib/Low-Pressure Blocks/Resistive Pipe LP  cs_type=1  d_in=station_3.pipe_diameter mm  area=1e-04 m^2  D_h=0.0112 m  s_factor=64  length=station_3.pipe_length_1 m  length_ad=1 m  roughness=0.005 mm  Re_lam=2e+03  Re_turb=4e+03  elevation_A=station_3.elevation m  elevation_B=station_3.elevation m  g=9.80665 m/s^2  pressure_drop_specify=off  pressure_drop_priority=None  pressure_drop=0 Pa  pressure_drop_nominal_specify=off  pressure_drop_nominal_unit=Pa  pressure_drop_nominal_value=1  flow_rate_specify=off  flow_rate_priority=None  flow_rate=0 m^3/s  flow_rate_nominal_specify=off  flow_rate_nominal_unit=m^3/s  flow_rate_nominal_value=1
      settings: SourceProductName=Simscape Fluids  SourceProductBaseCode=SH
  Pump 1 : sh_lib/Pumps and Motors/Centrifugal Pump  mdl_type=2  c_1=326.8 Pa/(kg/m^3)  c_2=3.104e+04 Pa*s/kg  c_3=1.097e+07 Pa*s^2/(kg*m^3)  c_4=2.136e+05 Pa*s^2/(kg*m^3)  c_f=0.8  design_del=130 lpm  ref_velocity=1.77e+03 rpm  ref_density=1000 kg/m^3  leak_resistance=1e+8 Pa/(m^3/s)  T_const=0.1 N*m  trq_press_coeff=1e-6 N*m/Pa  pump_del_1D=pump_3.Q m^3/s  press_diff_1D=pump_3.P bar  pump_del_power_1D=pump_3.Q m^3/s  power_1D=pump_3.N W  pump_vel_2D="[  3.2e+03 3.3e+03 3.4e+03 3.5e+03 ] rpm"  pump_del_2D="[  0 50 100 150 200 250 300 350 ] lpm"  press_diff_2D="[  8.3 8.8 9.3 9.9 ; 7.8 8.3 8.8 9.4 ; 7.2 7.6 8.2 8.7 ; 6.5 7 7.5 8 ; 5.6 6.1 6.6 7.1 ; 4.7 5.2 5.7 6.2 ; 3.4 4 4.4 4.9 ; 2.3 2.7 3.4 3.6 ; ] bar"  pump_del_power_2D="[  0 50 100 150 200 250 300 350 ] lpm"  power_2D="[  1.223e+03 1.341e+03 1.467e+03 1.6e+03 ; 1.414e+03 1.551e+03 1.696e+03 1.85e+03 ; 1.636e+03 1.794e+03 1.962e+03 2.14e+03 ; 1.941e+03 2.129e+03 2.326e+03 2.54e+03 ; 2.224e+03 2.439e+03 2.66e+03 2.91e+03 ; 2.453e+03 2.691e+03 2.947e+03 3.21e+03 ; 2.757e+03 3.024e+03 3.307e+03 3.608e+03 ; 2.945e+03 3.23e+03 3.533e+03 3.854e+03 ; ] W"  omega_threshold=1e-9 rad/s  interp_method=2  extrap_method=1
      settings: SourceProductName=Simscape Fluids  SourceProductBaseCode=SH
  Pump 2 : sh_lib/Pumps and Motors/Centrifugal Pump  mdl_type=2  c_1=326.8 Pa/(kg/m^3)  c_2=3.104e+04 Pa*s/kg  c_3=1.097e+07 Pa*s^2/(kg*m^3)  c_4=2.136e+05 Pa*s^2/(kg*m^3)  c_f=0.8  design_del=130 lpm  ref_velocity=1.77e+03 rpm  ref_density=1000 kg/m^3  leak_resistance=1e+8 Pa/(m^3/s)  T_const=0.1 N*m  trq_press_coeff=1e-6 N*m/Pa  pump_del_1D=pump_3.Q m^3/s  press_diff_1D=pump_3.P bar  pump_del_power_1D=pump_3.Q m^3/s  power_1D=pump_3.N W  pump_vel_2D="[  3.2e+03 3.3e+03 3.4e+03 3.5e+03 ] rpm"  pump_del_2D="[  0 50 100 150 200 250 300 350 ] lpm"  press_diff_2D="[  8.3 8.8 9.3 9.9 ; 7.8 8.3 8.8 9.4 ; 7.2 7.6 8.2 8.7 ; 6.5 7 7.5 8 ; 5.6 6.1 6.6 7.1 ; 4.7 5.2 5.7 6.2 ; 3.4 4 4.4 4.9 ; 2.3 2.7 3.4 3.6 ; ] bar"  pump_del_power_2D="[  0 50 100 150 200 250 300 350 ] lpm"  power_2D="[  1.223e+03 1.341e+03 1.467e+03 1.6e+03 ; 1.414e+03 1.551e+03 1.696e+03 1.85e+03 ; 1.636e+03 1.794e+03 1.962e+03 2.14e+03 ; 1.941e+03 2.129e+03 2.326e+03 2.54e+03 ; 2.224e+03 2.439e+03 2.66e+03 2.91e+03 ; 2.453e+03 2.691e+03 2.947e+03 3.21e+03 ; 2.757e+03 3.024e+03 3.307e+03 3.608e+03 ; 2.945e+03 3.23e+03 3.533e+03 3.854e+03 ; ] W"  omega_threshold=1e-9 rad/s  interp_method=2  extrap_method=1
      settings: SourceProductName=Simscape Fluids  SourceProductBaseCode=SH
  Simulink-PS Converter : nesl_utility/Simulink-PS Converter  PhysicalDomain=network_engine_domain  SubClassName=ps_input  LeftPortType=input  RightPortType=output  PseudoPeriodic=off  Frequencies=[]  NoiseDistribution=none  NoiseParameters=[]  Unit=rpm  AffineConversion=off  FilteringAndDerivatives=zero  SimscapeFilterOrder=1  InputFilterTimeConstant=.001  UdotUserProvided=0
  Simulink-PS Converter1 : nesl_utility/Simulink-PS Converter  PhysicalDomain=network_engine_domain  SubClassName=ps_input  LeftPortType=input  RightPortType=output  PseudoPeriodic=off  Frequencies=[]  NoiseDistribution=none  NoiseParameters=[]  Unit=rpm  AffineConversion=off  FilteringAndDerivatives=zero  SimscapeFilterOrder=1  InputFilterTimeConstant=.001  UdotUserProvided=0
  Speed Pump 1 : Constant  Value=1700
  Speed Pump 2 : Constant  Value=1700
  Velocity Source Pump 1 : fl_lib/Mechanical/Mechanical Sources/Ideal Angular Velocity Source
  Velocity Source Pump 2 : fl_lib/Mechanical/Mechanical Sources/Ideal Angular Velocity Source
  P : PMIOPort  Side=Right
  T : PMIOPort  Port=2  Side=Left
  wires:
  Speed Pump 2/1 -> Simulink-PS Converter/1
  Speed Pump 1/1 -> Simulink-PS Converter1/1
  connections:
  Velocity Source Pump 2/LConn1 -- Pump 2/LConn1
  Pump 1/RConn1 -- Pipe Pump 1P/LConn1
  Pump 1/RConn2 -- Pipe Pump 1T/RConn1
  Pump 2/RConn2 -- Pipe Pump 2T/RConn1
  T/RConn1 -- Pipe T/LConn1
  Pump 2/RConn1 -- Pipe Pump 2P/LConn1
  Pipe Pump 2T/LConn1 -- Pipe Pump 1T/LConn1 -- Pipe T/RConn1
  Simulink-PS Converter/RConn1 -- Velocity Source Pump 2/RConn1
  MRRef Pump 2/LConn1 -- Velocity Source Pump 2/RConn2
  Pipe Pump 1P/RConn1 -- Pipe Pump 2P/RConn1 -- Pipe P/LConn1
  P/RConn1 -- Pipe P/RConn1
  Simulink-PS Converter1/RConn1 -- Velocity Source Pump 1/RConn1
  MRRef Pump 1/LConn1 -- Velocity Source Pump 1/RConn2
  Velocity Source Pump 1/LConn1 -- Pump 1/LConn1

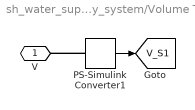
== system sh_water_supply_system/Volume T1 ==
  PS-Simulink Converter1 : nesl_utility/PS-Simulink Converter  PhysicalDomain=network_engine_domain  SubClassName=ps_output  LeftPortType=input  RightPortType=output  PseudoPeriodic=off  Frequencies=[]  Unit=1  AffineConversion=off
  V : PMIOPort  Side=Left
  tag scope: V_S1=global
  wires:
  PS-Simulink Converter1/1 -> [V_S1]
  connections:
  PS-Simulink Converter1/LConn1 -- V/RConn1

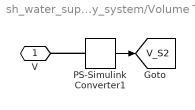
== system sh_water_supply_system/Volume T2 ==
  PS-Simulink Converter1 : nesl_utility/PS-Simulink Converter  PhysicalDomain=network_engine_domain  SubClassName=ps_output  LeftPortType=input  RightPortType=output  PseudoPeriodic=off  Frequencies=[]  Unit=1  AffineConversion=off
  V : PMIOPort  Side=Left
  tag scope: V_S2=global
  wires:
  PS-Simulink Converter1/1 -> [V_S2]
  connections:
  PS-Simulink Converter1/LConn1 -- V/RConn1

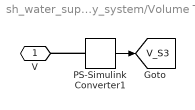
== system sh_water_supply_system/Volume T3 ==
  PS-Simulink Converter1 : nesl_utility/PS-Simulink Converter  PhysicalDomain=network_engine_domain  SubClassName=ps_output  LeftPortType=input  RightPortType=output  PseudoPeriodic=off  Frequencies=[]  Unit=1  AffineConversion=off
  V : PMIOPort  Side=Left
  tag scope: V_S3=global
  wires:
  PS-Simulink Converter1/1 -> [V_S3]
  connections:
  PS-Simulink Converter1/LConn1 -- V/RConn1

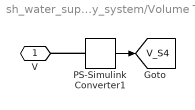
== system sh_water_supply_system/Volume T4 ==
  PS-Simulink Converter1 : nesl_utility/PS-Simulink Converter  PhysicalDomain=network_engine_domain  SubClassName=ps_output  LeftPortType=input  RightPortType=output  PseudoPeriodic=off  Frequencies=[]  Unit=1  AffineConversion=off
  V : PMIOPort  Side=Left
  tag scope: V_S4=global
  wires:
  PS-Simulink Converter1/1 -> [V_S4]
  connections:
  PS-Simulink Converter1/LConn1 -- V/RConn1
